simulink model "PLL__2"  (R2015a)
settings: Solver=ode45  StartTime=0.0  StopTime=10.0  RelTol=1e-3
values from neighbouring files (symbols this model uses):
  G0 = 1e3    (= 1000)    [PLL_1.m]    (also in PLL_2.m; PLL_3.m)
  K0 = 11.7    [PLL_2.m]    (also in PLL_3.m)
  N = 10    [PLL_1.m]    (also in PLL_2.m; PLL_3.m)
  RC = 2e-4    (= 0.0002)    [PLL_1.m]    (also in PLL_2.m; PLL_3.m)
  tau = 5e-5    (= 5e-05)    [PLL_1.m]    (also in PLL_2.m; PLL_3.m)
  Vm = 10    [PLL_1.m]    (also in PLL_2.m; PLL_3.m)
  w1 = 4.67e3    (= 4670)    [PLL_2.m]    (also in PLL_3.m)
  w2 = 21.4e3    (= 21400)    [PLL_2.m]    (also in PLL_3.m)
settings Model: Creator=mserrari  LastModifiedBy=mserrari

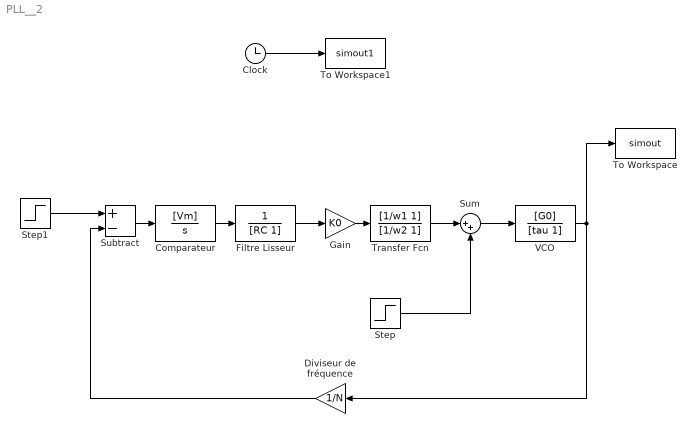
== system PLL__2 ==
  Clock : Clock
  Comparateur : TransferFcn  Numerator=[Vm]  Denominator=[1 0]
  Diviseur de fréquence : Gain  Gain=1/N
  Filtre Lisseur : TransferFcn  Denominator=[RC 1]
  Gain : Gain  Gain=K0
  Step : Step  Time=5  After=0.5  SampleTime=0
  Step1 : Step  After=10000  SampleTime=0
  Subtract : Sum  Inputs=+-
  Sum : Sum  Inputs=|++
  To Workspace : ToWorkspace  VariableName=simout  SaveFormat=Timeseries  SampleTime=-1
  To Workspace1 : ToWorkspace  VariableName=simout1  SaveFormat=Timeseries  SampleTime=-1
  Transfer Fcn : TransferFcn  Numerator=[1/w1 1]  Denominator=[1/w2 1]
  VCO : TransferFcn  Numerator=[G0]  Denominator=[tau 1]
  wires:
  Filtre Lisseur/1 -> Gain/1
  Comparateur/1 -> Filtre Lisseur/1
  VCO/1 -> To Workspace/1, Diviseur de fréquence/1
  Diviseur de fréquence/1 -> Subtract/2
  Subtract/1 -> Comparateur/1
  Step1/1 -> Subtract/1
  Gain/1 -> Transfer Fcn/1
  Sum/1 -> VCO/1
  Transfer Fcn/1 -> Sum/1
  Step/1 -> Sum/2
  Clock/1 -> To Workspace1/1
